simulink model "SimpleStateObserver"  (R2024b)
settings: Solver=VariableStepAuto  StartTime=0.0  StopTime=10.0  RelTol=1e-3
values from neighbouring files (symbols this model uses):
  C = Ts/(Tc+Ts)    [Simple_observer.m]
  denLPF = [Tc, Ts-Tc]    [Simple_observer.m]
  denSpeedFilter = [1,0,0,0]    [Simple_observer.m]
  numLPF = [Ts]    [Simple_observer.m]
  numSpeedFilter = 1/(N*Ts)*[1,0,0,-1]    [Simple_observer.m]
  Ts = 1e-2    (= 0.01)    [balrob_params.m]
undefined symbols (not defined in the file or in its folder): DiscIntNeverNeededParam, gbox, sens
settings Model: Creator=llp  LastModifiedBy=Davide Pillon

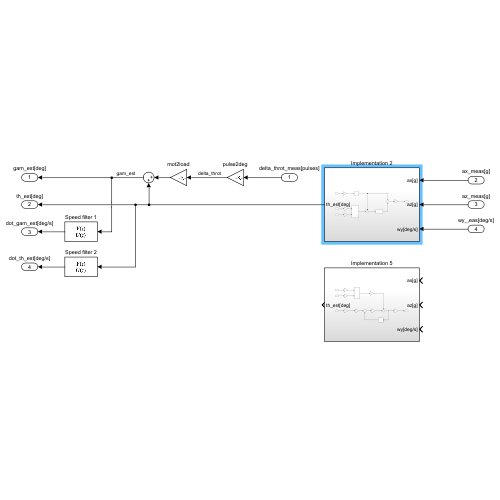
[thumbnail: Simulink's stored preview of the top-level diagram]
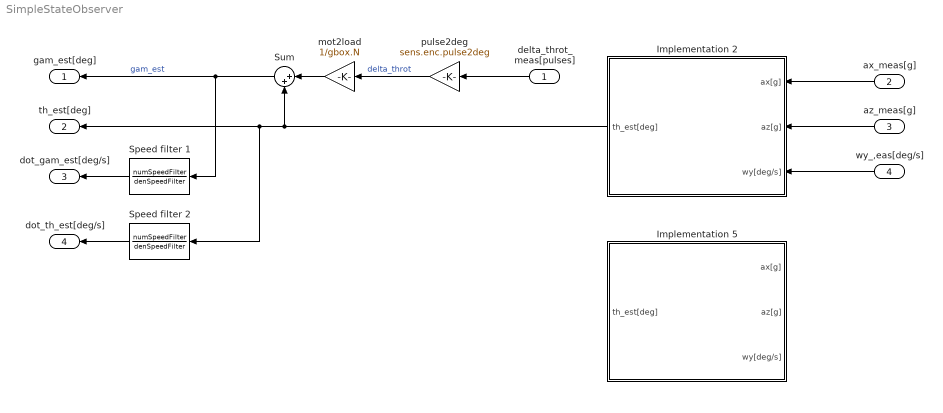
== system SimpleStateObserver ==
  delta_throt_meas[pulses] : Inport
  ax_meas[g] : Inport  Port=2
  az_meas[g] : Inport  Port=3
  wy_,eas[deg/s] : Inport  Port=4
  Implementation 2 : Subsystem
  Implementation 5 : Subsystem
  Speed filter 1 : DiscreteTransferFcn  Numerator=numSpeedFilter  Denominator=denSpeedFilter
  Speed filter 2 : DiscreteTransferFcn  Numerator=numSpeedFilter  Denominator=denSpeedFilter
  Sum : Sum  Inputs=|++
  mot2load : Gain  Gain=1/gbox.N
  pulse2deg : Gain  Gain=sens.enc.pulse2deg
  gam_est[deg] : Outport
  th_est[deg] : Outport  Port=2
  dot_gam_est[deg/s] : Outport  Port=3
  dot_th_est[deg/s] : Outport  Port=4
  wires:
  delta_throt_meas[pulses]/1 -> pulse2deg/1
  pulse2deg/1 -> mot2load/1  "delta_throt"
  mot2load/1 -> Sum/1
  Sum/1 -> Speed filter 1/1, gam_est[deg]/1  "gam_est"
  Speed filter 2/1 -> dot_th_est[deg/s]/1
  Speed filter 1/1 -> dot_gam_est[deg/s]/1
  Implementation 2/1(th_est[deg]) -> Sum/2, th_est[deg]/1, Speed filter 2/1
  ax_meas[g]/1 -> Implementation 2/1(ax[g])
  az_meas[g]/1 -> Implementation 2/2(az[g])
  wy_,eas[deg/s]/1 -> Implementation 2/3(wy[deg/s])

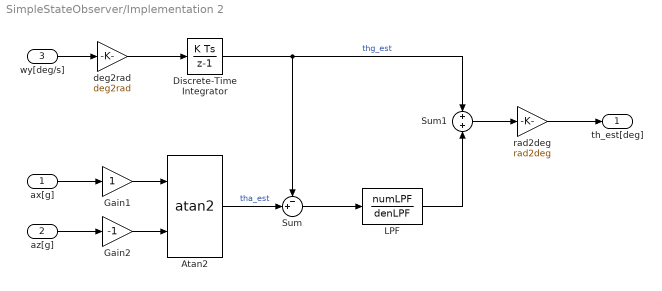
== system SimpleStateObserver/Implementation 2 ==
  ax[g] : Inport
  az[g] : Inport  Port=2
  wy[deg/s] : Inport  Port=3
  Atan2 : Trigonometry  Operator=atan2
  Discrete-Time Integrator : DiscreteIntegrator  SampleTime=Ts  ICPrevOutput=DiscIntNeverNeededParam  ICPrevScaledInput=DiscIntNeverNeededParam
  Gain1 : Gain
  Gain2 : Gain  Gain=-1
  LPF : DiscreteTransferFcn  Numerator=numLPF  Denominator=denLPF
  Sum : Sum  Inputs=-+|
  Sum1 : Sum
  deg2rad : Gain  Gain=deg2rad
  rad2deg : Gain  Gain=rad2deg
  th_est[deg] : Outport
  wires:
  wy[deg/s]/1 -> deg2rad/1
  ax[g]/1 -> Gain1/1
  az[g]/1 -> Gain2/1
  Gain1/1 -> Atan2/1
  Gain2/1 -> Atan2/2
  Atan2/1 -> Sum/2  "tha_est"
  deg2rad/1 -> Discrete-Time Integrator/1
  Discrete-Time Integrator/1 -> Sum1/1, Sum/1  "thg_est"
  rad2deg/1 -> th_est[deg]/1
  Sum1/1 -> rad2deg/1
  Sum/1 -> LPF/1
  LPF/1 -> Sum1/2

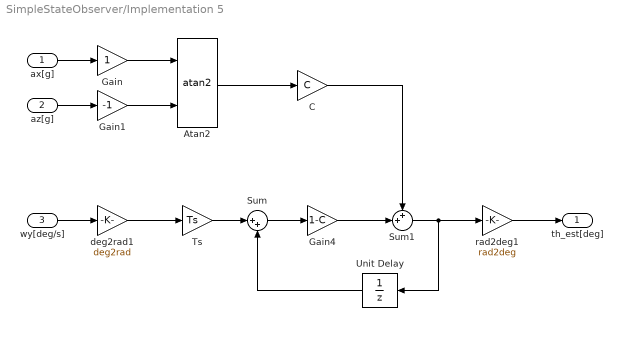
== system SimpleStateObserver/Implementation 5 ==
  ax[g] : Inport
  az[g] : Inport  Port=2
  wy[deg/s] : Inport  Port=3
  Atan2 : Trigonometry  Operator=atan2
  C : Gain  Gain=C
  Gain : Gain
  Gain1 : Gain  Gain=-1
  Gain4 : Gain  Gain=1-C
  Sum : Sum  Inputs=|++
  Sum1 : Sum  Inputs=++|
  Ts : Gain  Gain=Ts
  Unit Delay : UnitDelay  SampleTime=-1  HasFrameUpgradeWarning=on
  deg2rad1 : Gain  Gain=deg2rad
  rad2deg1 : Gain  Gain=rad2deg
  th_est[deg] : Outport
  wires:
  ax[g]/1 -> Gain/1
  az[g]/1 -> Gain1/1
  wy[deg/s]/1 -> deg2rad1/1
  deg2rad1/1 -> Ts/1
  Ts/1 -> Sum/1
  Sum/1 -> Gain4/1
  Unit Delay/1 -> Sum/2
  Gain4/1 -> Sum1/2
  Sum1/1 -> Unit Delay/1, rad2deg1/1
  rad2deg1/1 -> th_est[deg]/1
  Gain/1 -> Atan2/1
  Gain1/1 -> Atan2/2
  Atan2/1 -> C/1
  C/1 -> Sum1/1
